simulink model "CartesianImpedanceCtrlForUse"  (R2024a)
settings: Solver=ode45  StartTime=0.0  StopTime=tEnd+7  RelTol=1e-3
values from neighbouring files (symbols this model uses):
  Kf_gain = 100    [helperDesignImpedanceControl.m]
  neuromeka = importrobot(robotFile, DataFormat="column")    [helperDesignImpedanceControl.m]
  objectPos = 0.2    [helperDesignImpedanceControl.m]
  p_surface = [-0.30; -0.20; 0.35]    [helperDesignImpedanceControl.m]
  q_init = q_nmpc    [helperDesignImpedanceControl.m]
  tEnd = 5    [helperDesignImpedanceControl.m]
  Ts = 0.001    [helperDesignImpedanceControl.m]
  tStart = 0.5    [helperDesignImpedanceControl.m]
  use_force_feedback = 1    [helperDesignImpedanceControl.m]
undefined symbols (not defined in the file or in its folder): X, Y, Z
libraries: sm_lib x88, nesl_utility x54, matrix_library x4, robotcorelib x2, robotmaniplib x2, simulink x1
(part 1 of 3)
settings Model: PacingRate=0.450000  Creator=tshifera  LastModifiedBy=adekoyoa
settings RTWCC: GPUComputeCapability=3.5

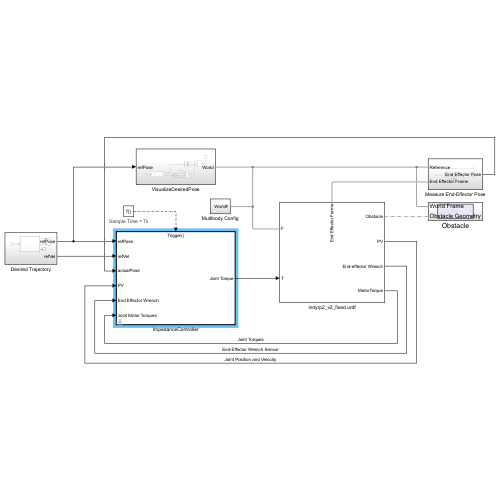
[thumbnail: Simulink's stored preview of the top-level diagram]
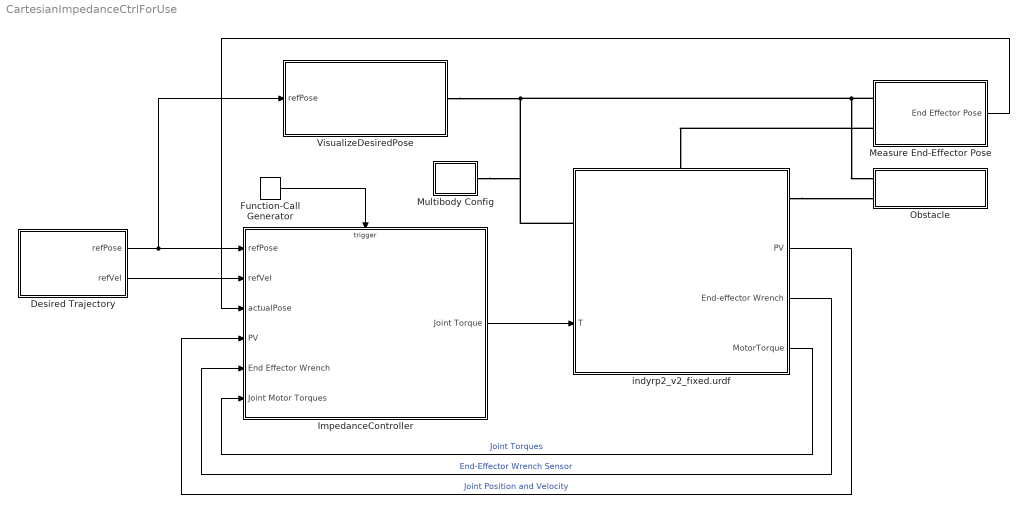
== system CartesianImpedanceCtrlForUse ==
  Desired Trajectory : Subsystem
  Function-Call Generator : simulink/Ports & Subsystems/Function-Call Generator  sample_time=Ts  numberOfIterations=1  DisallowWideOutput=off
      settings: AttributesFormatString=Sample Time = %<sample_time>
  ImpedanceController : Subsystem  mask(Impedance Controller for robotic arm){robot=neuromeka, Kd=diag([4 9 4 4 1 1 1]), Kt=100*eye(3), Ko=500*eye(3), Kc=50*eye(3)}
      mask prompts: robot "Robot (must be a rigidBodyTree object)"; Kd "Stabilizing joint damping, Kd (diag matrix, size is number of joints)"; Kt "Translational stiffness symmetric  matrix, Kt (3x3)"; Ko "Rotational stiffness symmetric  matrix, Ko (3x3)"; Kc "Coupling stiffness symmetric matrix, Kc (3x3)"
      mask help: Impedance control is a type of indirect force control at which we do not specify the forces to be applied by end-effector. Instead the interaction between the end-effector and environment is modeled as spring-mass-damper system. The impedance control aims to minimize contact forces between the end-effector and environment (object).
      mask init:
      | Go = calcCoStiffness(Ko); 
      | Gc = calcCoStiffness(Kc); 
      | Gt = calcCoStiffness(Kt);
      mask DialogControl Container3 Prompt: Mass-spring-damper system for Impedance Control, at End Effector position
  Measure End-Effector Pose : Subsystem
  Multibody Config : Subsystem
  Obstacle : Subsystem
  VisualizeDesiredPose : Subsystem
  indyrp2_v2_fixed.urdf : Subsystem
      settings: PortSchema="{\"entries\":[{\"content\":{\"sides\":[{\"content\":{\"connectorIds\":[\"LConn1\",\"In1\"]},\"type\":\"ConnectorPlacement.EquallySpacedRectSide\",\"uuid\":\"20be0e61-bde3-4ad2-a2a9-5f76c8900bc2\"},{\"content\":{\"connectorIds\":[\"RConn1\",\"Out1\",\"Out2\",\"Out3\"],\"side\":\"RIGHT\"},\"type\":\"ConnectorPlacement.EquallySpacedRectSide\",\"uuid\":\"1dd2584f-a73a-4303-a33e-8b83e7317fe8\"},{\"content\":{\"connectorIds\":[\"LConn2\"],\"side\":\"TOP\"},\"type\":\"ConnectorPlacement.EquallySpacedRectSide\",\"uuid\":\"0ecb7f5a-7207-4171-888d-c034677c21c8\"}]},\"type\":\"ConnectorPlacement.EquallySpacedConnector\",\"uuid\":\"de8f8f88-db56-4656-bd14-0e31f1d98c2e\"}],\"packageUris\":[\"http://schema.mathworks.com/mf0/Connector/R2020b\"],\"version\":\"1.0\"}"
  wires:
  ImpedanceController/1(Joint Torque) -> indyrp2_v2_fixed.urdf/1(T)
  indyrp2_v2_fixed.urdf/2(End-effector Wrench) -> ImpedanceController/5(End Effector Wrench)  "End-Effector Wrench Sensor"
  Function-Call Generator/1 -> ImpedanceController/Trigger
  Desired Trajectory/1(refPose) -> ImpedanceController/1(refPose), VisualizeDesiredPose/1(refPose)
  indyrp2_v2_fixed.urdf/3(MotorTorque) -> ImpedanceController/6(Joint Motor Torques)  "Joint Torques"
  indyrp2_v2_fixed.urdf/1(PV) -> ImpedanceController/4(PV)  "Joint Position and Velocity"
  Measure End-Effector Pose/1(End Effector Pose) -> ImpedanceController/3(actualPose)
  Desired Trajectory/2(refVel) -> ImpedanceController/2(refVel)
  connections:
  Measure End-Effector Pose/LConn1 -- Multibody Config/RConn1 -- indyrp2_v2_fixed.urdf/LConn1 -- VisualizeDesiredPose/RConn1 -- Obstacle/LConn1
  Measure End-Effector Pose/LConn2 -- indyrp2_v2_fixed.urdf/LConn2
  indyrp2_v2_fixed.urdf/RConn1 -- Obstacle/LConn2

== system CartesianImpedanceCtrlForUse/Desired Trajectory ==
  Clock : Clock
  Desired Transform Trajectory : robotcorelib/Transform Trajectory  WaypointSource=Internal  T0=task_init  TF=task_goal  TimeInterval=[tStart,tEnd]  CustomTimeScaling=off  ParameterSource=Internal  TSTime=2:0.1:3  TimeScaling=[ 0:0.1:1; ones( 1, 11 ); zeros( 1, 11 ) ]  SimulateUsing=Code generation
      settings: AttributesFormatString=|
      | Initial transform: %<T0>
      | Final transform: %<TF>
      | Time interval: %<TimeInterval>
  Terminator1 : Terminator
  refPose : Outport
  refVel : Outport  Port=2
  wires:
  Desired Transform Trajectory/3 -> Terminator1/1
  Desired Transform Trajectory/1 -> refPose/1
  Clock/1 -> Desired Transform Trajectory/1
  Desired Transform Trajectory/2 -> refVel/1

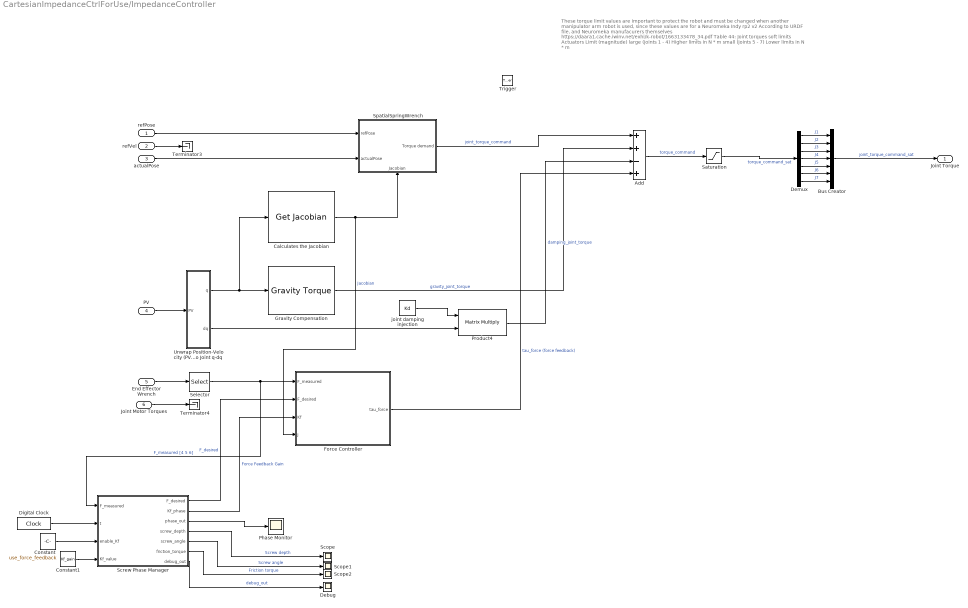
== system CartesianImpedanceCtrlForUse/ImpedanceController ==
  note: These torque limit values are important to protect the robot and must be changed when another manipulator arm robot is used, since these values are for a Neuromeka Indy rp2 v2
      |
      | According to URDF file, and Neuromeka manufacurers themselves
      | https://daara1.cache.iwinv.net/exhi/k-robot/1663133478_34.pdf
      | Table 44: Joint torques soft limits
      | Actuators Limit (magnitude)
      | large (joints 1 - 4) Higher limits in N * m
      | small (joints 5 - 7) Lower limits in N * m
  refPose : Inport
  refVel : Inport  Port=2
  actualPose : Inport  Port=3
  PV : Inport  Port=4
  End Effector Wrench : Inport  Port=5
  Joint Motor Torques : Inport  Port=6
  Trigger : TriggerPort  TriggerType=function-call  VariantControl=(inherit)  PortDimensions=1
  Add : Sum  Inputs=++-+
  Bus Creator : BusCreator  Inputs=7
  Calculates the Jacobian : robotmaniplib/Get Jacobian  RigidBodyTree=robot  EndEffector=tcp  SimulateUsing=Code generation
  Constant : Constant  Value=use_force_feedback
  Constant1 : Constant  Value=Kf_gain
  Debug : Scope
  Demux : Demux  Outputs=7
  Digital Clock : DigitalClock  SampleTime=-1
  Force Controller : MATLAB Function  TreatAsAtomicUnit=on
  Gravity Compensation : robotmaniplib/Gravity Torque  RigidBodyTree=robot  SimulateUsing=Code generation
  Phase Monitor : Scope
  Product4 : Product  Multiplication=Matrix(*)
  Saturation : Saturate  UpperLimit=[431.97; 431.97; 197.23; 197.23; 79.79; 79.79; 79.79]  LowerLimit=-[431.97; 431.97; 197.23; 197.23; 79.79; 79.79; 79.79]
      settings: AttributesFormatString=|
      | LowerLimit: %<LowerLimit>
      | UpperLimit: %<UpperLimit>
  Scope : Scope
  Scope1 : Scope
  Scope2 : Scope
  Screw Phase Manager : MATLAB Function  TreatAsAtomicUnit=on
  Selector : Selector  InputPortWidth=6  IndexOptions=Index vector (dialog)  Indices=[4 5 6]  OutputSizes=1
  SpatialSpringWrench : Subsystem
      settings: PortSchema="{\"entries\":[{\"content\":{\"sides\":[{\"content\":{\"connectorIds\":[\"In1\",\"In2\"]},\"type\":\"ConnectorPlacement.EquallySpacedRectSide\",\"uuid\":\"87e22711-7bf7-4371-9005-a78890a45407\"},{\"content\":{\"connectorIds\":[\"Out1\"],\"side\":\"RIGHT\"},\"type\":\"ConnectorPlacement.EquallySpacedRectSide\",\"uuid\":\"305db76c-9102-4628-bb77-ff13562ba12d\"},{\"content\":{\"connectorIds\":[],\"side\":\"TOP\"},\"type\":\"ConnectorPlacement.EquallySpacedRectSide\",\"uuid\":\"789cf5b2-3cb1-4c2b-9242-fa29b46ec439\"},{\"content\":{\"connectorIds\":[\"In3\"],\"side\":\"BOTTOM\"},\"type\":\"ConnectorPlacement.EquallySpacedRectSide\",\"uuid\":\"eb4e7ef0-db2a-4ad3-a69c-cad197a1a56b\"}]},\"type\":\"ConnectorPlacement.EquallySpacedConnector\",\"uuid\":\"6ecf40e4-a298-4160-8c5e-e2bf95d6c265\"}],\"packageUris\":[\"http://schema.mathworks.com/mf0/Connector/R2020b\"],\"version\":\"1.0\"}"
  Terminator3 : Terminator
  Terminator4 : Terminator
  Unwrap Position-Velocity (PV) to Joint q-dq : Subsystem
  joint damping injection : Constant  Value=Kd
  Joint Torque : Outport
  wires:
  End Effector Wrench/1 -> Selector/1
  Unwrap Position-Velocity (PV) to Joint q-dq/2(dq) -> Product4/2
  Unwrap Position-Velocity (PV) to Joint q-dq/1(q) -> Calculates the Jacobian/1, Gravity Compensation/1
  Joint Motor Torques/1 -> Terminator4/1
  refVel/1 -> Terminator3/1
  Product4/1 -> Add/3  "damping_joint_torque"
  PV/1 -> Unwrap Position-Velocity (PV) to Joint q-dq/1(PV)
  actualPose/1 -> SpatialSpringWrench/2(actualPose)
  Saturation/1 -> Demux/1  "torque_command_sat"
  Bus Creator/1 -> Joint Torque/1  "joint_torque_command_sat"
  SpatialSpringWrench/1(Torque demand) -> Add/1  "joint_torque_command"
  Calculates the Jacobian/1 -> SpatialSpringWrench/3(Jacobian), Force Controller/4(J)  "Jacobian"
  Gravity Compensation/1 -> Add/2  "gravity_joint_torque"
  Add/1 -> Saturation/1  "torque_command"
  Demux/2 -> Bus Creator/2  "J2"
  Demux/7 -> Bus Creator/7  "J7"
  Demux/3 -> Bus Creator/3  "J3"
  Demux/4 -> Bus Creator/4  "J4"
  Demux/6 -> Bus Creator/6  "J6"
  Demux/5 -> Bus Creator/5  "J5"
  refPose/1 -> SpatialSpringWrench/1(refPose)
  Demux/1 -> Bus Creator/1  "J1"
  joint damping injection/1 -> Product4/1
  Selector/1 -> Force Controller/1(F_measured), Screw Phase Manager/1(F_measured)  "F_measured [4 5 6]"
  Screw Phase Manager/1(F_desired) -> Force Controller/2(F_desired)  "F_desired"
  Screw Phase Manager/2(Kf_phase) -> Force Controller/3(Kf)  "Force Feedback Gain"
  Force Controller/1(tau_force) -> Add/4  "tau_force (force feedback)"
  Screw Phase Manager/3(phase_out) -> Phase Monitor/1
  Digital Clock/1 -> Screw Phase Manager/2(t)
  Screw Phase Manager/4(screw_depth) -> Scope/1  "Screw depth"
  Screw Phase Manager/5(screw_angle) -> Scope1/1  "Screw angle"
  Screw Phase Manager/6(friction_torque) -> Scope2/1  "Friction torque"
  Screw Phase Manager/7(debug_out) -> Debug/1  "debug_out"
  Constant1/1 -> Screw Phase Manager/4(Kf_value)
  Constant/1 -> Screw Phase Manager/3(enable_Kf)

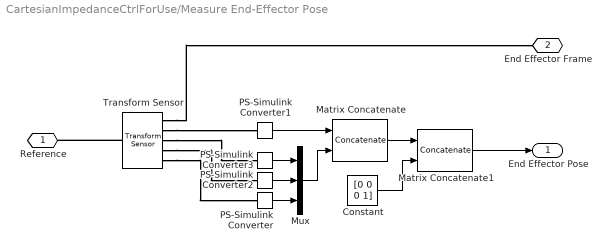
== system CartesianImpedanceCtrlForUse/Measure End-Effector Pose ==
  Constant : Constant  Value=[0 0 0 1]  VectorParams1D=off
  Matrix Concatenate : Concatenate  Mode=Multidimensional array  ConcatenateDimension=2
  Matrix Concatenate1 : Concatenate  Mode=Multidimensional array
  Mux : Mux  Inputs=3
  PS-Simulink Converter{,1..3} (4 alike) : nesl_utility/PS-Simulink Converter  PhysicalDomain=network_engine_domain  SubClassName=ps_output  LeftPortType=input  RightPortType=output  PseudoPeriodic=off  Frequencies=[]  VectorFormat=inherit  Unit=inherit  AffineConversion=off
  Transform Sensor : sm_lib/Frames and Transforms/Transform Sensor  MeasurementFrame=World  RotationSequence=XYX  SenseAngle=off  SenseAxis=off  SenseQ=off  SenseR=on  SenseRotationSequence=off  SenseOmegaX=off  SenseOmegaY=off  SenseOmegaZ=off  SenseOmega=off  SenseQDot=off  SenseRDot=off  SenseRotationSequenceDot=off  SenseAlphaX=off  SenseAlphaY=off  SenseAlphaZ=off  SenseAlpha=off  SenseQDDot=off  SenseRDDot=off  SenseX=on  SenseY=on  SenseZ=on  SenseXYZ=off  SenseRad=off  SenseAzim=off  SenseDist=off  SenseInc=off  SenseXDot=off  SenseYDot=off  SenseZDot=off  SenseXYZDot=off  SenseRadDot=off  SenseAzimDot=off  SenseDistDot=off  SenseIncDot=off  SenseXDDot=off  SenseYDDot=off  SenseZDDot=off  SenseXYZDDot=off  SenseRadDDot=off  SenseAzimDDot=off  SenseDistDDot=off  SenseIncDDot=off
  Reference : PMIOPort  Side=Left
  End Effector Frame : PMIOPort  Port=2  Side=Left
  End Effector Pose : Outport
  wires:
  PS-Simulink Converter2/1 -> Mux/2
  PS-Simulink Converter1/1 -> Matrix Concatenate/1
  Constant/1 -> Matrix Concatenate1/2
  Matrix Concatenate/1 -> Matrix Concatenate1/1
  Mux/1 -> Matrix Concatenate/2
  PS-Simulink Converter/1 -> Mux/3
  PS-Simulink Converter3/1 -> Mux/1
  Matrix Concatenate1/1 -> End Effector Pose/1
  connections:
  Transform Sensor/RConn2 -- PS-Simulink Converter1/LConn1
  Transform Sensor/RConn3 -- PS-Simulink Converter3/LConn1
  Transform Sensor/RConn5 -- PS-Simulink Converter/LConn1
  Transform Sensor/RConn4 -- PS-Simulink Converter2/LConn1
  Transform Sensor/LConn1 -- Reference/RConn1
  Transform Sensor/RConn1 -- End Effector Frame/RConn1

== system CartesianImpedanceCtrlForUse/Multibody Config ==
  MechanismConfiguration : sm_lib/Utilities/Mechanism Configuration  UniformGravity=Constant  GravityVector=neuromeka.Gravity  GravityVectorUnits=m/s^2  LinearizationDelta=0.001  JointModeTransitionNonlinearIterations=2
  Solver Configuration : nesl_utility/Solver Configuration  PhysicalDomain=network_engine_domain  SubClassName=solver  LeftPortType=input  RightPortType=generic  Tones=[]  Harmonics=[]  SimulateNoise=off  Profile=off  UseLocalSampling=off  EnableSwitchedLinearOptims=on  FrequencyDomain=off  UseCCode=off  RelTol=0.001  AbsTol=0.001  MinStep=1e-09  ToWorkspace=off  RevertToSquareIcSolve=off  NumHomotopyIterations=100  PhasorMode=off  PhasorModeNumHarmonics=1  ConsistencySolver=NEWTON_FTOL  IndexReductionMethod=DerivativeReplacement  DoDC=off  ResidualTolerance=1e-09  ConsistencyTolSource=GLOBAL  ConsistencyAbsTol=0.001  ConsistencyRelTol=0.001  ConsistencyTolFactor=0.001  UseLocalSolver=off  LocalSolverChoice=NE_BACKWARD_EULER_ADVANCER  ResolveIndetEquations=on  FunctionEvalNumThread=1  LocalSolverSampleTime=0.001  DoFixedCost=off  MaxNonlinIter=3  MaxModeIter=2  ComputeImpulses=off  ImpulseIterations=2  LinearAlgebra=auto  LinearAlgebraNumThread=0  EquationFormulation=NE_TIME_EF  DelaysMemoryBudget=1024  AutomaticFiltering=on  FilteringTimeConstant=0.001  PartitionStorageMethod=AS_NEEDED  PartitionMemoryBudget=1024  PartitionMethod=ROBUST  MultibodyUseLocalSolver=off  MultibodyLocalSolverChoice=ODE1  MultibodyLocalSolverSampleTime=0.001
  World : sm_lib/Frames and Transforms/World Frame
  WorldF : PMIOPort  Side=Right
  connections:
  MechanismConfiguration/RConn1 -- WorldF/RConn1 -- World/RConn1 -- Solver Configuration/RConn1

== system CartesianImpedanceCtrlForUse/Obstacle ==
  note: Obstacle object
  Cartesian Joint : sm_lib/Joints/Cartesian Joint  JointMode=Normal  CompositeWrenchDir=FollowerOnBase  CompositeWrenchFrame=BaseFrame  SenseConstraintForce=off  SenseConstraintTorque=off  SenseTotalForce=off  SenseTotalTorque=off  PxPositionTargetSpecify=on  PxPositionTargetPriority=High  PxPositionTargetValue=-0.3  PxPositionTargetValueUnits=m  PxVelocityTargetSpecify=off  PxVelocityTargetPriority=High  PxVelocityTargetValue=0  PxVelocityTargetValueUnits=m/s  PxEquilibriumPosition=0  PxEquilibriumPositionUnits=m  PxSpringStiffness=0  PxSpringStiffnessUnits=N/m  PxDampingCoefficient=0  PxDampingCoefficientUnits=N/(m/s)  PxLowerLimitSpecify=off  PxLowerLimitBound=-1  PxLowerLimitBoundUnits=m  PxLowerLimitStiffness=1e6  PxLowerLimitStiffnessUnits=N/m  PxLowerLimitDamping=1e3  PxLowerLimitDampingUnits=N/(m/s)  PxLowerLimitTransitionRegionWidth=1e-4  PxLowerLimitTransitionRegionWidthUnits=m  PxUpperLimitSpecify=off  PxUpperLimitBound=1  PxUpperLimitBoundUnits=m  PxUpperLimitStiffness=1e6  PxUpperLimitStiffnessUnits=N/m  PxUpperLimitDamping=1e3  PxUpperLimitDampingUnits=N/(m/s)  PxUpperLimitTransitionRegionWidth=1e-4  PxUpperLimitTransitionRegionWidthUnits=m  PxTorqueActuationMode=ComputedTorque  PxMotionActuationMode=InputMotion  PxSensePosition=off  PxSenseVelocity=off  PxSenseAcceleration=off  PxSenseTorqueForce=off  PxSenseLowerLimitTorqueForce=off  PxSenseUpperLimitTorqueForce=off  PyPositionTargetSpecify=on  PyPositionTargetPriority=High  PyPositionTargetValue=-0.2  PyPositionTargetValueUnits=m  PyVelocityTargetSpecify=off  PyVelocityTargetPriority=High  PyVelocityTargetValue=0  PyVelocityTargetValueUnits=m/s  PyEquilibriumPosition=0  PyEquilibriumPositionUnits=m  PySpringStiffness=0  PySpringStiffnessUnits=N/m  PyDampingCoefficient=0  PyDampingCoefficientUnits=N/(m/s)  PyLowerLimitSpecify=off  PyLowerLimitBound=-1  PyLowerLimitBoundUnits=m  PyLowerLimitStiffness=1e6  PyLowerLimitStiffnessUnits=N/m  PyLowerLimitDamping=1e3  PyLowerLimitDampingUnits=N/(m/s)  PyLowerLimitTransitionRegionWidth=1e-4  PyLowerLimitTransitionRegionWidthUnits=m  PyUpperLimitSpecify=off  PyUpperLimitBound=1  PyUpperLimitBoundUnits=m  PyUpperLimitStiffness=1e6  PyUpperLimitStiffnessUnits=N/m  PyUpperLimitDamping=1e3  PyUpperLimitDampingUnits=N/(m/s)  PyUpperLimitTransitionRegionWidth=1e-4  PyUpperLimitTransitionRegionWidthUnits=m  PyTorqueActuationMode=NoTorque  PyMotionActuationMode=ComputedMotion  PySensePosition=off  PySenseVelocity=off  PySenseAcceleration=off  PySenseTorqueForce=off  PySenseLowerLimitTorqueForce=off  PySenseUpperLimitTorqueForce=off  PzPositionTargetSpecify=on  PzPositionTargetPriority=High  PzPositionTargetValue=0.2  PzPositionTargetValueUnits=m  PzVelocityTargetSpecify=off  PzVelocityTargetPriority=High  PzVelocityTargetValue=0  PzVelocityTargetValueUnits=m/s  PzEquilibriumPosition=0  PzEquilibriumPositionUnits=m  PzSpringStiffness=0  PzSpringStiffnessUnits=N/m  PzDampingCoefficient=0  PzDampingCoefficientUnits=N/(m/s)  PzLowerLimitSpecify=off  PzLowerLimitBound=-1  PzLowerLimitBoundUnits=m  PzLowerLimitStiffness=1e6  PzLowerLimitStiffnessUnits=N/m  PzLowerLimitDamping=1e3  PzLowerLimitDampingUnits=N/(m/s)  PzLowerLimitTransitionRegionWidth=1e-4  PzLowerLimitTransitionRegionWidthUnits=m  PzUpperLimitSpecify=off  PzUpperLimitBound=1  PzUpperLimitBoundUnits=m  PzUpperLimitStiffness=1e6  PzUpperLimitStiffnessUnits=N/m  PzUpperLimitDamping=1e3  PzUpperLimitDampingUnits=N/(m/s)  PzUpperLimitTransitionRegionWidth=1e-4  PzUpperLimitTransitionRegionWidthUnits=m  PzTorqueActuationMode=ComputedTorque  PzMotionActuationMode=InputMotion  PzSensePosition=off  PzSenseVelocity=off  PzSenseAcceleration=off  PzSenseTorqueForce=off  PzSenseLowerLimitTorqueForce=off  PzSenseUpperLimitTorqueForce=off
  Constant : Constant  Value=objectPos
  Constant2 : Constant  Value=p_surface(1)
  Simulink-PS Converter7 : nesl_utility/Simulink-PS Converter  PhysicalDomain=network_engine_domain  SubClassName=ps_input  LeftPortType=input  RightPortType=output  PseudoPeriodic=off  Frequencies=[]  NoiseDistribution=none  NoiseParameters=[]  Unit=1  AffineConversion=off  FilteringAndDerivatives=filter  SimscapeFilterOrder=2  InputFilterTimeConstant=1e-2  UdotUserProvided=0
  Simulink-PS Converter8 : nesl_utility/Simulink-PS Converter  PhysicalDomain=network_engine_domain  SubClassName=ps_input  LeftPortType=input  RightPortType=output  PseudoPeriodic=off  Frequencies=[]  NoiseDistribution=none  NoiseParameters=[]  Unit=1  AffineConversion=off  FilteringAndDerivatives=provide  SimscapeFilterOrder=2  InputFilterTimeConstant=0.001  UdotUserProvided=0
  Wall Object : Subsystem
  World Frame : PMIOPort  Side=Left
  Obstacle Geometry : PMIOPort  Port=2  Side=Left
  tag scope: ObstaclePos=global
  wires:
  Constant2/1 -> Simulink-PS Converter8/1
  Constant/1 -> Simulink-PS Converter7/1, [ObstaclePos]  "obstacle Position"
  connections:
  World Frame/RConn1 -- Cartesian Joint/LConn1
  Wall Object/RConn1 -- Obstacle Geometry/RConn1
  Simulink-PS Converter7/RConn1 -- Cartesian Joint/LConn3
  Simulink-PS Converter8/RConn1 -- Cartesian Joint/LConn2
  Wall Object/LConn1 -- Cartesian Joint/RConn1

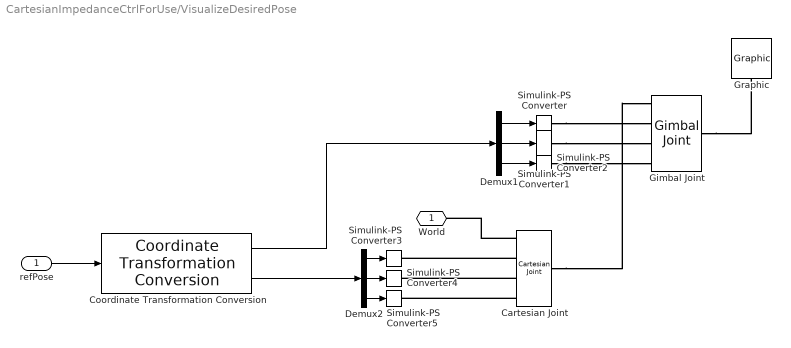
== system CartesianImpedanceCtrlForUse/VisualizeDesiredPose ==
  refPose : Inport
  Cartesian Joint : sm_lib/Joints/Cartesian Joint  JointMode=Normal  CompositeWrenchDir=FollowerOnBase  CompositeWrenchFrame=BaseFrame  SenseConstraintForce=off  SenseConstraintTorque=off  SenseTotalForce=off  SenseTotalTorque=off  PxPositionTargetSpecify=off  PxPositionTargetPriority=High  PxPositionTargetValue=0  PxPositionTargetValueUnits=m  PxVelocityTargetSpecify=off  PxVelocityTargetPriority=High  PxVelocityTargetValue=0  PxVelocityTargetValueUnits=m/s  PxEquilibriumPosition=0  PxEquilibriumPositionUnits=m  PxSpringStiffness=0  PxSpringStiffnessUnits=N/m  PxDampingCoefficient=0  PxDampingCoefficientUnits=N/(m/s)  PxLowerLimitSpecify=off  PxLowerLimitBound=-1  PxLowerLimitBoundUnits=m  PxLowerLimitStiffness=1e6  PxLowerLimitStiffnessUnits=N/m  PxLowerLimitDamping=1e3  PxLowerLimitDampingUnits=N/(m/s)  PxLowerLimitTransitionRegionWidth=1e-4  PxLowerLimitTransitionRegionWidthUnits=m  PxUpperLimitSpecify=off  PxUpperLimitBound=1  PxUpperLimitBoundUnits=m  PxUpperLimitStiffness=1e6  PxUpperLimitStiffnessUnits=N/m  PxUpperLimitDamping=1e3  PxUpperLimitDampingUnits=N/(m/s)  PxUpperLimitTransitionRegionWidth=1e-4  PxUpperLimitTransitionRegionWidthUnits=m  PxTorqueActuationMode=ComputedTorque  PxMotionActuationMode=InputMotion  PxSensePosition=off  PxSenseVelocity=off  PxSenseAcceleration=off  PxSenseTorqueForce=off  PxSenseLowerLimitTorqueForce=off  PxSenseUpperLimitTorqueForce=off  PyPositionTargetSpecify=off  PyPositionTargetPriority=High  PyPositionTargetValue=0  PyPositionTargetValueUnits=m  PyVelocityTargetSpecify=off  PyVelocityTargetPriority=High  PyVelocityTargetValue=0  PyVelocityTargetValueUnits=m/s  PyEquilibriumPosition=0  PyEquilibriumPositionUnits=m  PySpringStiffness=0  PySpringStiffnessUnits=N/m  PyDampingCoefficient=0  PyDampingCoefficientUnits=N/(m/s)  PyLowerLimitSpecify=off  PyLowerLimitBound=-1  PyLowerLimitBoundUnits=m  PyLowerLimitStiffness=1e6  PyLowerLimitStiffnessUnits=N/m  PyLowerLimitDamping=1e3  PyLowerLimitDampingUnits=N/(m/s)  PyLowerLimitTransitionRegionWidth=1e-4  PyLowerLimitTransitionRegionWidthUnits=m  PyUpperLimitSpecify=off  PyUpperLimitBound=1  PyUpperLimitBoundUnits=m  PyUpperLimitStiffness=1e6  PyUpperLimitStiffnessUnits=N/m  PyUpperLimitDamping=1e3  PyUpperLimitDampingUnits=N/(m/s)  PyUpperLimitTransitionRegionWidth=1e-4  PyUpperLimitTransitionRegionWidthUnits=m  PyTorqueActuationMode=ComputedTorque  PyMotionActuationMode=InputMotion  PySensePosition=off  PySenseVelocity=off  PySenseAcceleration=off  PySenseTorqueForce=off  PySenseLowerLimitTorqueForce=off  PySenseUpperLimitTorqueForce=off  PzPositionTargetSpecify=off  PzPositionTargetPriority=High  PzPositionTargetValue=0  PzPositionTargetValueUnits=m  PzVelocityTargetSpecify=off  PzVelocityTargetPriority=High  PzVelocityTargetValue=0  PzVelocityTargetValueUnits=m/s  PzEquilibriumPosition=0  PzEquilibriumPositionUnits=m  PzSpringStiffness=0  PzSpringStiffnessUnits=N/m  PzDampingCoefficient=0  PzDampingCoefficientUnits=N/(m/s)  PzLowerLimitSpecify=off  PzLowerLimitBound=-1  PzLowerLimitBoundUnits=m  PzLowerLimitStiffness=1e6  PzLowerLimitStiffnessUnits=N/m  PzLowerLimitDamping=1e3  PzLowerLimitDampingUnits=N/(m/s)  PzLowerLimitTransitionRegionWidth=1e-4  PzLowerLimitTransitionRegionWidthUnits=m  PzUpperLimitSpecify=off  PzUpperLimitBound=1  PzUpperLimitBoundUnits=m  PzUpperLimitStiffness=1e6  PzUpperLimitStiffnessUnits=N/m  PzUpperLimitDamping=1e3  PzUpperLimitDampingUnits=N/(m/s)  PzUpperLimitTransitionRegionWidth=1e-4  PzUpperLimitTransitionRegionWidthUnits=m  PzTorqueActuationMode=ComputedTorque  PzMotionActuationMode=InputMotion  PzSensePosition=off  PzSenseVelocity=off  PzSenseAcceleration=off  PzSenseTorqueForce=off  PzSenseLowerLimitTorqueForce=off  PzSenseUpperLimitTorqueForce=off
  Coordinate Transformation Conversion : robotcorelib/Coordinate Transformation Conversion  InputRepresentation=Homogeneous Transformation  InputEulerSequence=ZYX  ShowTrVecInputPort=on  OutputRepresentation=Euler Angles  OutputEulerSequence=XYZ  ShowTrVecOutputPort=on  SimulateUsing=Interpreted execution
  Demux1 : Demux  Outputs=3
  Demux2 : Demux  Outputs=3
  Gimbal Joint : sm_lib/Joints/Gimbal Joint  JointMode=Normal  CompositeWrenchDir=FollowerOnBase  CompositeWrenchFrame=BaseFrame  SenseConstraintForce=off  SenseConstraintTorque=off  SenseTotalForce=off  SenseTotalTorque=off  RxPositionTargetSpecify=off  RxPositionTargetPriority=High  RxPositionTargetValue=0  RxPositionTargetValueUnits=deg  RxVelocityTargetSpecify=off  RxVelocityTargetPriority=High  RxVelocityTargetValue=0  RxVelocityTargetValueUnits=deg/s  RxEquilibriumPosition=0  RxEquilibriumPositionUnits=deg  RxSpringStiffness=0  RxSpringStiffnessUnits=N*m/deg  RxDampingCoefficient=0  RxDampingCoefficientUnits=N*m/(deg/s)  RxLowerLimitSpecify=off  RxLowerLimitBound=-90  RxLowerLimitBoundUnits=deg  RxLowerLimitStiffness=1e4  RxLowerLimitStiffnessUnits=N*m/deg  RxLowerLimitDamping=10  RxLowerLimitDampingUnits=N*m/(deg/s)  RxLowerLimitTransitionRegionWidth=0.1  RxLowerLimitTransitionRegionWidthUnits=deg  RxUpperLimitSpecify=off  RxUpperLimitBound=90  RxUpperLimitBoundUnits=deg  RxUpperLimitStiffness=1e4  RxUpperLimitStiffnessUnits=N*m/deg  RxUpperLimitDamping=10  RxUpperLimitDampingUnits=N*m/(deg/s)  RxUpperLimitTransitionRegionWidth=0.1  RxUpperLimitTransitionRegionWidthUnits=deg  RxTorqueActuationMode=ComputedTorque  RxMotionActuationMode=InputMotion  RxSensePosition=off  RxSenseVelocity=off  RxSenseAcceleration=off  RxSenseTorqueForce=off  RxSenseLowerLimitTorqueForce=off  RxSenseUpperLimitTorqueForce=off  RyPositionTargetSpecify=off  RyPositionTargetPriority=High  RyPositionTargetValue=0  RyPositionTargetValueUnits=deg  RyVelocityTargetSpecify=off  RyVelocityTargetPriority=High  RyVelocityTargetValue=0  RyVelocityTargetValueUnits=deg/s  RyEquilibriumPosition=0  RyEquilibriumPositionUnits=deg  RySpringStiffness=0  RySpringStiffnessUnits=N*m/deg  RyDampingCoefficient=0  RyDampingCoefficientUnits=N*m/(deg/s)  RyLowerLimitSpecify=off  RyLowerLimitBound=-90  RyLowerLimitBoundUnits=deg  RyLowerLimitStiffness=1e4  RyLowerLimitStiffnessUnits=N*m/deg  RyLowerLimitDamping=10  RyLowerLimitDampingUnits=N*m/(deg/s)  RyLowerLimitTransitionRegionWidth=0.1  RyLowerLimitTransitionRegionWidthUnits=deg  RyUpperLimitSpecify=off  RyUpperLimitBound=90  RyUpperLimitBoundUnits=deg  RyUpperLimitStiffness=1e4  RyUpperLimitStiffnessUnits=N*m/deg  RyUpperLimitDamping=10  RyUpperLimitDampingUnits=N*m/(deg/s)  RyUpperLimitTransitionRegionWidth=0.1  RyUpperLimitTransitionRegionWidthUnits=deg  RyTorqueActuationMode=ComputedTorque  RyMotionActuationMode=InputMotion  RySensePosition=off  RySenseVelocity=off  RySenseAcceleration=off  RySenseTorqueForce=off  RySenseLowerLimitTorqueForce=off  RySenseUpperLimitTorqueForce=off  RzPositionTargetSpecify=off  RzPositionTargetPriority=High  RzPositionTargetValue=0  RzPositionTargetValueUnits=deg  RzVelocityTargetSpecify=off  RzVelocityTargetPriority=High  RzVelocityTargetValue=0  RzVelocityTargetValueUnits=deg/s  RzEquilibriumPosition=0  RzEquilibriumPositionUnits=deg  RzSpringStiffness=0  RzSpringStiffnessUnits=N*m/deg  RzDampingCoefficient=0  RzDampingCoefficientUnits=N*m/(deg/s)  RzLowerLimitSpecify=off  RzLowerLimitBound=-90  RzLowerLimitBoundUnits=deg  RzLowerLimitStiffness=1e4  RzLowerLimitStiffnessUnits=N*m/deg  RzLowerLimitDamping=10  RzLowerLimitDampingUnits=N*m/(deg/s)  RzLowerLimitTransitionRegionWidth=0.1  RzLowerLimitTransitionRegionWidthUnits=deg  RzUpperLimitSpecify=off  RzUpperLimitBound=90  RzUpperLimitBoundUnits=deg  RzUpperLimitStiffness=1e4  RzUpperLimitStiffnessUnits=N*m/deg  RzUpperLimitDamping=10  RzUpperLimitDampingUnits=N*m/(deg/s)  RzUpperLimitTransitionRegionWidth=0.1  RzUpperLimitTransitionRegionWidthUnits=deg  RzTorqueActuationMode=ComputedTorque  RzMotionActuationMode=InputMotion  RzSensePosition=off  RzSenseVelocity=off  RzSenseAcceleration=off  RzSenseTorqueForce=off  RzSenseLowerLimitTorqueForce=off  RzSenseUpperLimitTorqueForce=off
  Graphic : sm_lib/Body Elements/Graphic  GraphicType=Marker  MarkerShape=Sphere  MarkerSize=15  GraphicVisPropType=SimpleVisualProperties  GraphicDiffuseColor=[1 0 0]  GraphicOpacity=1.0  GraphicSpecularColor=[0.5 0.5 0.5 1.0]  GraphicAmbientColor=[0.15 0.15 0.15 1.0]  GraphicEmissiveColor=[0.0 0.0 0.0 1.0]  GraphicShininess=75
  Simulink-PS Converter{,2..5} (5 alike) : nesl_utility/Simulink-PS Converter  PhysicalDomain=network_engine_domain  SubClassName=ps_input  LeftPortType=input  RightPortType=output  PseudoPeriodic=off  Frequencies=[]  NoiseDistribution=none  NoiseParameters=[]  Unit=1  AffineConversion=off  FilteringAndDerivatives=filter  SimscapeFilterOrder=2  InputFilterTimeConstant=0.001  UdotUserProvided=0
  Simulink-PS Converter1 : nesl_utility/Simulink-PS Converter  PhysicalDomain=network_engine_domain  SubClassName=ps_input  LeftPortType=input  RightPortType=output  PseudoPeriodic=off  Frequencies=[]  NoiseDistribution=none  NoiseParameters=[]  Unit=1  AffineConversion=off  FilteringAndDerivatives=filter  SimscapeFilterOrder=2  InputFilterTimeConstant=0.001  UdotUserProvided=1
  World : PMIOPort  Side=Right
  wires:
  Demux2/2 -> Simulink-PS Converter4/1
  Demux2/3 -> Simulink-PS Converter5/1
  Demux1/3 -> Simulink-PS Converter2/1
  Coordinate Transformation Conversion/1 -> Demux1/1
  Demux2/1 -> Simulink-PS Converter3/1
  Demux1/1 -> Simulink-PS Converter/1
  Demux1/2 -> Simulink-PS Converter1/1
  Coordinate Transformation Conversion/2 -> Demux2/1
  refPose/1 -> Coordinate Transformation Conversion/1
  connections:
  Cartesian Joint/LConn2 -- Simulink-PS Converter3/RConn1
  Cartesian Joint/RConn1 -- Gimbal Joint/LConn1
  Cartesian Joint/LConn3 -- Simulink-PS Converter4/RConn1
  Simulink-PS Converter1/RConn1 -- Gimbal Joint/LConn3
  Simulink-PS Converter/RConn1 -- Gimbal Joint/LConn2
  Cartesian Joint/LConn4 -- Simulink-PS Converter5/RConn1
  Simulink-PS Converter2/RConn1 -- Gimbal Joint/LConn4
  Gimbal Joint/RConn1 -- Graphic/RConn1
  Cartesian Joint/LConn1 -- World/RConn1

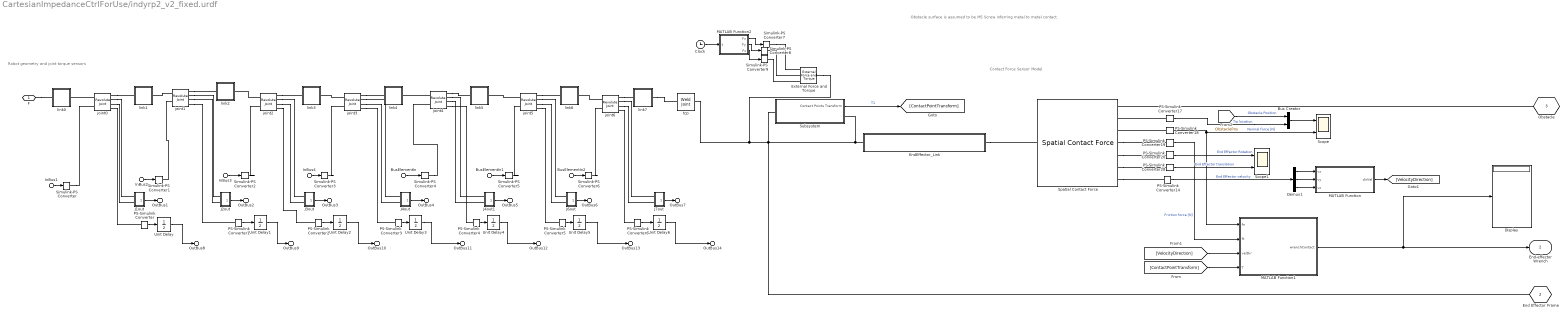
== system CartesianImpedanceCtrlForUse/indyrp2_v2_fixed.urdf ==
  note: Obstacle surface is assumed to be M5 Screw inferring metal to metal contact.
  note: Robot geometry and joint torque sensors
  note: Contact Force Sensor Model
  InBus1 : Inport  PortName=T  Element=J1
  InBus2 : Inport  PortName=T  Element=J2
  InBus3 : Inport  PortName=T  Element=J3
  InBus4 : Inport  PortName=T  Element=J4
  BusElementIn : Inport  PortName=T  Element=J5
  BusElementIn1 : Inport  PortName=T  Element=J6
  BusElementIn2 : Inport  PortName=T  Element=J7
  Bus Creator : BusCreator  Inputs=2
  Clock : Clock
  Demux1 : Demux  Outputs=3
  Display : Display
  EndEffector_Link : Subsystem
  External Force and Torque : sm_lib/Forces and Torques/External Force and Torque  EnableForceX=on  EnableForceY=on  EnableForceZ=on  EnableForce=off  ForceResolutionFrame=AttachedFrame  EnableTorqueX=off  EnableTorqueY=off  EnableTorqueZ=off  EnableTorque=off  TorqueResolutionFrame=AttachedFrame
  J1out : Subsystem
  J2out : Subsystem
  J3out : Subsystem
  J4out : Subsystem
  J4out1 : Subsystem
  J6out : Subsystem
  J7out : Subsystem
  MATLAB Function : MATLAB Function  TreatAsAtomicUnit=on
  MATLAB Function1 : MATLAB Function  TreatAsAtomicUnit=on
  MATLAB Function2 : MATLAB Function  TreatAsAtomicUnit=on
  PS-Simulink Converter{,1..6,14,17..20,28} (13 alike) : nesl_utility/PS-Simulink Converter  PhysicalDomain=network_engine_domain  SubClassName=ps_output  LeftPortType=input  RightPortType=output  PseudoPeriodic=off  Frequencies=[]  VectorFormat=inherit  Unit=inherit  AffineConversion=off
  Scope : Scope  NumInputPorts=2
  Scope1 : Scope  NumInputPorts=2
  Simulink-PS Converter{,1..6} (7 alike) : nesl_utility/Simulink-PS Converter  PhysicalDomain=network_engine_domain  SubClassName=ps_input  LeftPortType=input  RightPortType=output  PseudoPeriodic=off  Frequencies=[]  NoiseDistribution=none  NoiseParameters=[]  Unit=N*m  AffineConversion=off  FilteringAndDerivatives=provide  SimscapeFilterOrder=1  InputFilterTimeConstant=0.001  UdotUserProvided=0
  Simulink-PS Converter7 : nesl_utility/Simulink-PS Converter  PhysicalDomain=network_engine_domain  SubClassName=ps_input  LeftPortType=input  RightPortType=output  PseudoPeriodic=off  Frequencies=[]  NoiseDistribution=none  NoiseParameters=[]  Unit=1  AffineConversion=off  FilteringAndDerivatives=provide  SimscapeFilterOrder=1  InputFilterTimeConstant=0.001  UdotUserProvided=0
  Simulink-PS Converter8 : nesl_utility/Simulink-PS Converter  PhysicalDomain=network_engine_domain  SubClassName=ps_input  LeftPortType=input  RightPortType=output  PseudoPeriodic=off  Frequencies=[]  NoiseDistribution=none  NoiseParameters=[]  Unit=1  AffineConversion=off  FilteringAndDerivatives=provide  SimscapeFilterOrder=1  InputFilterTimeConstant=0.001  UdotUserProvided=0
  Simulink-PS Converter9 : nesl_utility/Simulink-PS Converter  PhysicalDomain=network_engine_domain  SubClassName=ps_input  LeftPortType=input  RightPortType=output  PseudoPeriodic=off  Frequencies=[]  NoiseDistribution=none  NoiseParameters=[]  Unit=1  AffineConversion=off  FilteringAndDerivatives=provide  SimscapeFilterOrder=1  InputFilterTimeConstant=0.001  UdotUserProvided=0
  Spatial Contact Force : sm_lib/Forces and Torques/Spatial Contact Force  NormalForceType=SmoothSpringDamper  NormalStiffness=K_contact  NormalStiffnessUnits=N/m  NormalDamping=D_contact  NormalDampingUnits=N/(m/s)  NormalTransitionRegionWidth=2  NormalTransitionRegionWidthUnits=mm  FrictionType=SmoothStickSlip  CoefficientOfStaticFriction=0.3  CoefficientOfDynamicFriction=0.2  FrictionalCriticalVelocity=1e-3  FrictionalCriticalVelocityUnits=m/s  SenseContactSignal=off  SensePenetrationDepth=off  SenseSeparationDistance=on  SenseNormalForceMagnitude=on  SenseFrictionalForceMagnitude=on  SenseNormalVelocity=on  SenseTangentialVelocity=off  SenseContactBaseRotation=on  SenseContactBaseTranslation=on  SenseContactFollowerRotation=off  SenseContactFollowerTranslation=off  ZeroCrossDetectContactStartAndEnd=off
      settings: AttributesFormatString=|
      | NormalStiffness = %<NormalStiffness> [%<NormalStiffnessUnits>]
      | NormalDamping = %<NormalDamping> [%<NormalDampingUnits>]
      | CoefficientOfStaticFriction = %<CoefficientOfStaticFriction>
      | CoefficientOfDynamicFriction = %<CoefficientOfDynamicFriction>
  Subsystem : Subsystem
  Unit Delay{,1..6} (7 alike) : UnitDelay  SampleTime=Ts  HasFrameUpgradeWarning=on
  joint0 : sm_lib/Joints/Revolute Joint  JointMode=Normal  CompositeWrenchDir=FollowerOnBase  CompositeWrenchFrame=BaseFrame  SenseConstraintForce=off  SenseConstraintTorque=off  SenseTotalForce=off  SenseTotalTorque=off  PositionTargetSpecify=on  PositionTargetPriority=High  PositionTargetValue=q_init(1)  PositionTargetValueUnits=rad  VelocityTargetSpecify=off  VelocityTargetPriority=High  VelocityTargetValue=0  VelocityTargetValueUnits=deg/s  EquilibriumPosition=0  EquilibriumPositionUnits=deg  SpringStiffness=0  SpringStiffnessUnits=N*m/deg  DampingCoefficient=0.1  DampingCoefficientUnits=kg*m^2/(rad*s)  LowerLimitSpecify=on  LowerLimitBound=-3.054326190990077  LowerLimitBoundUnits=rad  LowerLimitStiffness=1e4  LowerLimitStiffnessUnits=N*m/deg  LowerLimitDamping=10  LowerLimitDampingUnits=N*m/(deg/s)  LowerLimitTransitionRegionWidth=0.1  LowerLimitTransitionRegionWidthUnits=deg  UpperLimitSpecify=on  UpperLimitBound=3.054326190990077  UpperLimitBoundUnits=rad  UpperLimitStiffness=1e4  UpperLimitStiffnessUnits=N*m/deg  UpperLimitDamping=10  UpperLimitDampingUnits=N*m/(deg/s)  UpperLimitTransitionRegionWidth=0.1  UpperLimitTransitionRegionWidthUnits=deg  TorqueActuationMode=InputTorque  MotionActuationMode=ComputedMotion  SensePosition=on  SenseVelocity=on  SenseAcceleration=off  SenseTorqueForce=on  SenseLowerLimitTorqueForce=off  SenseUpperLimitTorqueForce=off
  joint1 : sm_lib/Joints/Revolute Joint  JointMode=Normal  CompositeWrenchDir=FollowerOnBase  CompositeWrenchFrame=BaseFrame  SenseConstraintForce=off  SenseConstraintTorque=off  SenseTotalForce=off  SenseTotalTorque=off  PositionTargetSpecify=on  PositionTargetPriority=High  PositionTargetValue=q_init(2)  PositionTargetValueUnits=deg  VelocityTargetSpecify=off  VelocityTargetPriority=High  VelocityTargetValue=0  VelocityTargetValueUnits=deg/s  EquilibriumPosition=0  EquilibriumPositionUnits=deg  SpringStiffness=0  SpringStiffnessUnits=N*m/deg  DampingCoefficient=0.1  DampingCoefficientUnits=kg*m^2/(rad*s)  LowerLimitSpecify=on  LowerLimitBound=-3.054326190990077  LowerLimitBoundUnits=rad  LowerLimitStiffness=1e4  LowerLimitStiffnessUnits=N*m/deg  LowerLimitDamping=10  LowerLimitDampingUnits=N*m/(deg/s)  LowerLimitTransitionRegionWidth=0.1  LowerLimitTransitionRegionWidthUnits=deg  UpperLimitSpecify=on  UpperLimitBound=3.054326190990077  UpperLimitBoundUnits=rad  UpperLimitStiffness=1e4  UpperLimitStiffnessUnits=N*m/deg  UpperLimitDamping=10  UpperLimitDampingUnits=N*m/(deg/s)  UpperLimitTransitionRegionWidth=0.1  UpperLimitTransitionRegionWidthUnits=deg  TorqueActuationMode=InputTorque  MotionActuationMode=ComputedMotion  SensePosition=on  SenseVelocity=on  SenseAcceleration=off  SenseTorqueForce=on  SenseLowerLimitTorqueForce=off  SenseUpperLimitTorqueForce=off
  joint2 : sm_lib/Joints/Revolute Joint  JointMode=Normal  CompositeWrenchDir=FollowerOnBase  CompositeWrenchFrame=BaseFrame  SenseConstraintForce=off  SenseConstraintTorque=off  SenseTotalForce=off  SenseTotalTorque=off  PositionTargetSpecify=on  PositionTargetPriority=High  PositionTargetValue=q_init(3)  PositionTargetValueUnits=deg  VelocityTargetSpecify=off  VelocityTargetPriority=High  VelocityTargetValue=0  VelocityTargetValueUnits=deg/s  EquilibriumPosition=0  EquilibriumPositionUnits=deg  SpringStiffness=0  SpringStiffnessUnits=N*m/deg  DampingCoefficient=0.1  DampingCoefficientUnits=kg*m^2/(rad*s)  LowerLimitSpecify=on  LowerLimitBound=-3.054326190990077  LowerLimitBoundUnits=rad  LowerLimitStiffness=1e4  LowerLimitStiffnessUnits=N*m/deg  LowerLimitDamping=10  LowerLimitDampingUnits=N*m/(deg/s)  LowerLimitTransitionRegionWidth=0.1  LowerLimitTransitionRegionWidthUnits=deg  UpperLimitSpecify=on  UpperLimitBound=3.054326190990077  UpperLimitBoundUnits=rad  UpperLimitStiffness=1e4  UpperLimitStiffnessUnits=N*m/deg  UpperLimitDamping=10  UpperLimitDampingUnits=N*m/(deg/s)  UpperLimitTransitionRegionWidth=0.1  UpperLimitTransitionRegionWidthUnits=deg  TorqueActuationMode=InputTorque  MotionActuationMode=ComputedMotion  SensePosition=on  SenseVelocity=on  SenseAcceleration=off  SenseTorqueForce=on  SenseLowerLimitTorqueForce=off  SenseUpperLimitTorqueForce=off
  joint3 : sm_lib/Joints/Revolute Joint  JointMode=Normal  CompositeWrenchDir=FollowerOnBase  CompositeWrenchFrame=BaseFrame  SenseConstraintForce=off  SenseConstraintTorque=off  SenseTotalForce=off  SenseTotalTorque=off  PositionTargetSpecify=on  PositionTargetPriority=High  PositionTargetValue=q_init(4)  PositionTargetValueUnits=deg  VelocityTargetSpecify=off  VelocityTargetPriority=High  VelocityTargetValue=0  VelocityTargetValueUnits=deg/s  EquilibriumPosition=0  EquilibriumPositionUnits=deg  SpringStiffness=0  SpringStiffnessUnits=N*m/deg  DampingCoefficient=0.1  DampingCoefficientUnits=kg*m^2/(rad*s)  LowerLimitSpecify=on  LowerLimitBound=-3.054326190990077  LowerLimitBoundUnits=rad  LowerLimitStiffness=1e4  LowerLimitStiffnessUnits=N*m/deg  LowerLimitDamping=10  LowerLimitDampingUnits=N*m/(deg/s)  LowerLimitTransitionRegionWidth=0.1  LowerLimitTransitionRegionWidthUnits=deg  UpperLimitSpecify=on  UpperLimitBound=3.054326190990077  UpperLimitBoundUnits=rad  UpperLimitStiffness=1e4  UpperLimitStiffnessUnits=N*m/deg  UpperLimitDamping=10  UpperLimitDampingUnits=N*m/(deg/s)  UpperLimitTransitionRegionWidth=0.1  UpperLimitTransitionRegionWidthUnits=deg  TorqueActuationMode=InputTorque  MotionActuationMode=ComputedMotion  SensePosition=on  SenseVelocity=on  SenseAcceleration=off  SenseTorqueForce=on  SenseLowerLimitTorqueForce=off  SenseUpperLimitTorqueForce=off
  joint4 : sm_lib/Joints/Revolute Joint  JointMode=Normal  CompositeWrenchDir=FollowerOnBase  CompositeWrenchFrame=BaseFrame  SenseConstraintForce=off  SenseConstraintTorque=off  SenseTotalForce=off  SenseTotalTorque=off  PositionTargetSpecify=on  PositionTargetPriority=High  PositionTargetValue=q_init(5)  PositionTargetValueUnits=deg  VelocityTargetSpecify=off  VelocityTargetPriority=High  VelocityTargetValue=0  VelocityTargetValueUnits=deg/s  EquilibriumPosition=0  EquilibriumPositionUnits=deg  SpringStiffness=0  SpringStiffnessUnits=N*m/deg  DampingCoefficient=0.1  DampingCoefficientUnits=kg*m^2/(rad*s)  LowerLimitSpecify=on  LowerLimitBound=-3.054326190990077  LowerLimitBoundUnits=rad  LowerLimitStiffness=1e4  LowerLimitStiffnessUnits=N*m/deg  LowerLimitDamping=10  LowerLimitDampingUnits=N*m/(deg/s)  LowerLimitTransitionRegionWidth=0.1  LowerLimitTransitionRegionWidthUnits=deg  UpperLimitSpecify=on  UpperLimitBound=3.054326190990077  UpperLimitBoundUnits=rad  UpperLimitStiffness=1e4  UpperLimitStiffnessUnits=N*m/deg  UpperLimitDamping=10  UpperLimitDampingUnits=N*m/(deg/s)  UpperLimitTransitionRegionWidth=0.1  UpperLimitTransitionRegionWidthUnits=deg  TorqueActuationMode=InputTorque  MotionActuationMode=ComputedMotion  SensePosition=on  SenseVelocity=on  SenseAcceleration=off  SenseTorqueForce=on  SenseLowerLimitTorqueForce=off  SenseUpperLimitTorqueForce=off
  joint5 : sm_lib/Joints/Revolute Joint  JointMode=Normal  CompositeWrenchDir=FollowerOnBase  CompositeWrenchFrame=BaseFrame  SenseConstraintForce=off  SenseConstraintTorque=off  SenseTotalForce=off  SenseTotalTorque=off  PositionTargetSpecify=on  PositionTargetPriority=High  PositionTargetValue=q_init(6)  PositionTargetValueUnits=deg  VelocityTargetSpecify=off  VelocityTargetPriority=High  VelocityTargetValue=0  VelocityTargetValueUnits=deg/s  EquilibriumPosition=0  EquilibriumPositionUnits=deg  SpringStiffness=0  SpringStiffnessUnits=N*m/deg  DampingCoefficient=0.1  DampingCoefficientUnits=kg*m^2/(rad*s)  LowerLimitSpecify=on  LowerLimitBound=-3.054326190990077  LowerLimitBoundUnits=rad  LowerLimitStiffness=1e4  LowerLimitStiffnessUnits=N*m/deg  LowerLimitDamping=10  LowerLimitDampingUnits=N*m/(deg/s)  LowerLimitTransitionRegionWidth=0.1  LowerLimitTransitionRegionWidthUnits=deg  UpperLimitSpecify=on  UpperLimitBound=3.054326190990077  UpperLimitBoundUnits=rad  UpperLimitStiffness=1e4  UpperLimitStiffnessUnits=N*m/deg  UpperLimitDamping=10  UpperLimitDampingUnits=N*m/(deg/s)  UpperLimitTransitionRegionWidth=0.1  UpperLimitTransitionRegionWidthUnits=deg  TorqueActuationMode=InputTorque  MotionActuationMode=ComputedMotion  SensePosition=on  SenseVelocity=on  SenseAcceleration=off  SenseTorqueForce=on  SenseLowerLimitTorqueForce=off  SenseUpperLimitTorqueForce=off
  joint6 : sm_lib/Joints/Revolute Joint  JointMode=Normal  CompositeWrenchDir=FollowerOnBase  CompositeWrenchFrame=BaseFrame  SenseConstraintForce=off  SenseConstraintTorque=off  SenseTotalForce=off  SenseTotalTorque=off  PositionTargetSpecify=on  PositionTargetPriority=High  PositionTargetValue=q_init(7)  PositionTargetValueUnits=deg  VelocityTargetSpecify=off  VelocityTargetPriority=High  VelocityTargetValue=0  VelocityTargetValueUnits=deg/s  EquilibriumPosition=0  EquilibriumPositionUnits=deg  SpringStiffness=0  SpringStiffnessUnits=N*m/deg  DampingCoefficient=0.1  DampingCoefficientUnits=kg*m^2/(rad*s)  LowerLimitSpecify=on  LowerLimitBound=-3.054326190990077  LowerLimitBoundUnits=rad  LowerLimitStiffness=1e4  LowerLimitStiffnessUnits=N*m/deg  LowerLimitDamping=10  LowerLimitDampingUnits=N*m/(deg/s)  LowerLimitTransitionRegionWidth=0.1  LowerLimitTransitionRegionWidthUnits=deg  UpperLimitSpecify=on  UpperLimitBound=3.054326190990077  UpperLimitBoundUnits=rad  UpperLimitStiffness=1e4  UpperLimitStiffnessUnits=N*m/deg  UpperLimitDamping=10  UpperLimitDampingUnits=N*m/(deg/s)  UpperLimitTransitionRegionWidth=0.1  UpperLimitTransitionRegionWidthUnits=deg  TorqueActuationMode=InputTorque  MotionActuationMode=ComputedMotion  SensePosition=on  SenseVelocity=on  SenseAcceleration=off  SenseTorqueForce=on  SenseLowerLimitTorqueForce=off  SenseUpperLimitTorqueForce=off
  link0 : Subsystem
  link1 : Subsystem
  link2 : Subsystem
  link3 : Subsystem
  link4 : Subsystem
  link5 : Subsystem
  link6 : Subsystem
  link7 : Subsystem
  tcp : sm_lib/Joints/Weld Joint  JointMode=Normal  CompositeWrenchDir=FollowerOnBase  CompositeWrenchFrame=BaseFrame  SenseConstraintForce=off  SenseConstraintTorque=off  SenseTotalForce=off  SenseTotalTorque=off
  F : PMIOPort  Side=Left
  End Effector Frame : PMIOPort  Port=2  Side=Left
  Obstacle : PMIOPort  Port=3  Side=Right
  OutBus1 : Outport  VectorParamsAs1DForOutWhenUnconnected=off  PortName=PV  Element=J1
  OutBus2 : Outport  VectorParamsAs1DForOutWhenUnconnected=off  PortName=PV  Element=J2
  OutBus3 : Outport  VectorParamsAs1DForOutWhenUnconnected=off  PortName=PV  Element=J3
  OutBus4 : Outport  VectorParamsAs1DForOutWhenUnconnected=off  PortName=PV  Element=J4
  OutBus5 : Outport  VectorParamsAs1DForOutWhenUnconnected=off  PortName=PV  Element=J5
  OutBus6 : Outport  VectorParamsAs1DForOutWhenUnconnected=off  PortName=PV  Element=J6
  OutBus7 : Outport  VectorParamsAs1DForOutWhenUnconnected=off  PortName=PV  Element=J7
  End-effector Wrench : Outport  Port=2
  OutBus8 : Outport  Port=3  VectorParamsAs1DForOutWhenUnconnected=off  PortName=MotorTorque  Element=J1
  OutBus9 : Outport  Port=3  VectorParamsAs1DForOutWhenUnconnected=off  PortName=MotorTorque  Element=J2
  OutBus10 : Outport  Port=3  VectorParamsAs1DForOutWhenUnconnected=off  PortName=MotorTorque  Element=J3
  OutBus11 : Outport  Port=3  VectorParamsAs1DForOutWhenUnconnected=off  PortName=MotorTorque  Element=J4
  OutBus12 : Outport  Port=3  VectorParamsAs1DForOutWhenUnconnected=off  PortName=MotorTorque  Element=J5
  OutBus13 : Outport  Port=3  VectorParamsAs1DForOutWhenUnconnected=off  PortName=MotorTorque  Element=J6
  OutBus14 : Outport  Port=3  VectorParamsAs1DForOutWhenUnconnected=off  PortName=MotorTorque  Element=J7
  wires:
  J4out/1(J4) -> OutBus4/1
  BusElementIn/1 -> Simulink-PS Converter4/1
  InBus4/1 -> Simulink-PS Converter3/1
  J7out/1(J7) -> OutBus7/1
  InBus1/1 -> Simulink-PS Converter/1
  InBus3/1 -> Simulink-PS Converter2/1
  InBus2/1 -> Simulink-PS Converter1/1
  J6out/1(J6) -> OutBus6/1
  J1out/1(J1) -> OutBus1/1
  J2out/1(J2) -> OutBus2/1
  J4out1/1(J5) -> OutBus5/1
  J3out/1(J3) -> OutBus3/1
  BusElementIn1/1 -> Simulink-PS Converter5/1
  BusElementIn2/1 -> Simulink-PS Converter6/1
  Subsystem/1(Contact Points Transform) -> [ContactPointTransform]  "T1"
  MATLAB Function1/1(wrenchContact) -> Display/1, End-effector Wrench/1
  PS-Simulink Converter20/1 -> Scope1/1  "End Effector Rotation"
  PS-Simulink Converter28/1 -> Scope1/2  "End Effector translation"
  PS-Simulink Converter18/1 -> Scope/2, MATLAB Function1/1(fn)  "Normal force [N]"
  [ContactPointTransform] -> MATLAB Function1/4(T)
  Demux1/1 -> MATLAB Function/1(vx)
  Demux1/3 -> MATLAB Function/3(vz)
  MATLAB Function/1(dirVel) -> [VelocityDirection]
  Demux1/2 -> MATLAB Function/2(vy)
  PS-Simulink Converter14/1 -> Demux1/1  "End Effector velocity"
  [VelocityDirection] -> MATLAB Function1/3(velDir)
  PS-Simulink Converter19/1 -> MATLAB Function1/2(ft)  "Friction force [N]"
  PS-Simulink Converter/1 -> Unit Delay/1
  PS-Simulink Converter1/1 -> Unit Delay1/1
  PS-Simulink Converter2/1 -> Unit Delay2/1
  PS-Simulink Converter3/1 -> Unit Delay3/1
  PS-Simulink Converter4/1 -> Unit Delay4/1
  PS-Simulink Converter5/1 -> Unit Delay5/1
  PS-Simulink Converter6/1 -> Unit Delay6/1
  Unit Delay/1 -> OutBus8/1
  Unit Delay1/1 -> OutBus9/1
  Unit Delay2/1 -> OutBus10/1
  Unit Delay3/1 -> OutBus11/1
  Unit Delay4/1 -> OutBus12/1
  Unit Delay5/1 -> OutBus13/1
  Unit Delay6/1 -> OutBus14/1
  PS-Simulink Converter17/1 -> Bus Creator/2  "Tip location"
  Bus Creator/1 -> Scope/1
  [ObstaclePos] -> Bus Creator/1  "Obstacle Position"
  Clock/1 -> MATLAB Function2/1(t)
  MATLAB Function2/1(Fx) -> Simulink-PS Converter7/1
  MATLAB Function2/2(Fy) -> Simulink-PS Converter8/1
  MATLAB Function2/3(Fz) -> Simulink-PS Converter9/1
  connections:
  Subsystem/RConn1 -- EndEffector_Link/LConn1 -- External Force and Torque/RConn1 -- tcp/RConn1 -- Subsystem/LConn1 -- End Effector Frame/RConn1
  PS-Simulink Converter18/LConn1 -- Spatial Contact Force/RConn3
  Spatial Contact Force/RConn5 -- PS-Simulink Converter20/LConn1
  Spatial Contact Force/RConn4 -- PS-Simulink Converter19/LConn1
  PS-Simulink Converter17/LConn1 -- Spatial Contact Force/RConn2
  Obstacle/RConn1 -- Spatial Contact Force/RConn1
  EndEffector_Link/RConn1 -- Spatial Contact Force/LConn1
  Spatial Contact Force/RConn7 -- PS-Simulink Converter14/LConn1
  Spatial Contact Force/RConn6 -- PS-Simulink Converter28/LConn1
  joint4/LConn1 -- link4/RConn1
  joint3/LConn1 -- link3/RConn1
  joint0/RConn1 -- link1/LConn1
  joint2/LConn1 -- link2/RConn1
  joint3/RConn1 -- link4/LConn1
  joint6/RConn1 -- link7/LConn1
  joint0/LConn1 -- link0/RConn1
  joint6/LConn1 -- link6/RConn1
  link7/RConn1 -- tcp/LConn1
  joint1/LConn1 -- link1/RConn1
  joint2/RConn1 -- link3/LConn1
  joint1/RConn1 -- link2/LConn1
  joint5/RConn1 -- link6/LConn1
  F/RConn1 -- link0/LConn1
  joint5/LConn1 -- link5/RConn1
  joint4/RConn1 -- link5/LConn1
  Simulink-PS Converter/RConn1 -- joint0/LConn2
  joint0/RConn2 -- J1out/LConn1
  joint0/RConn3 -- J1out/LConn2
  joint0/RConn4 -- PS-Simulink Converter/LConn1
  Simulink-PS Converter1/RConn1 -- joint1/LConn2
  joint1/RConn2 -- J2out/LConn1
  joint1/RConn3 -- J2out/LConn2
  joint1/RConn4 -- PS-Simulink Converter1/LConn1
  Simulink-PS Converter2/RConn1 -- joint2/LConn2
  joint2/RConn2 -- J3out/LConn1
  joint2/RConn3 -- J3out/LConn2
  joint2/RConn4 -- PS-Simulink Converter2/LConn1
  Simulink-PS Converter3/RConn1 -- joint3/LConn2
  joint3/RConn2 -- J4out/LConn1
  joint3/RConn3 -- J4out/LConn2
  joint3/RConn4 -- PS-Simulink Converter3/LConn1
  Simulink-PS Converter4/RConn1 -- joint4/LConn2
  joint4/RConn2 -- J4out1/LConn1
  joint4/RConn3 -- J4out1/LConn2
  joint4/RConn4 -- PS-Simulink Converter4/LConn1
  Simulink-PS Converter5/RConn1 -- joint5/LConn2
  joint5/RConn2 -- J6out/LConn1
  joint5/RConn3 -- J6out/LConn2
  joint5/RConn4 -- PS-Simulink Converter5/LConn1
  Simulink-PS Converter6/RConn1 -- joint6/LConn2
  joint6/RConn2 -- J7out/LConn1
  joint6/RConn3 -- J7out/LConn2
  joint6/RConn4 -- PS-Simulink Converter6/LConn1
  Simulink-PS Converter7/RConn1 -- External Force and Torque/LConn1
  Simulink-PS Converter8/RConn1 -- External Force and Torque/LConn2
  Simulink-PS Converter9/RConn1 -- External Force and Torque/LConn3
